simulink model "aBaja2026"  (R2025b)
settings: Solver=FixedStepAuto  StartTime=0  StopTime=1000  FixedStep=timeStep  RelTol=1e-3
PostLoadFcn:
  | helperSLTrajectoryFollowerWithRRScenarioSetup
InitFcn:
  | helperSLTrajectoryFollowerWithRRScenarioSetup
  | worldActor=rrSim.getScenario();
  | world = worldActor.actor_spec.world_spec;
  | % Inputs you already have (example):
  | EgoActorID  = 1;
  | egoSetSpeed = 0;
  | 
  | % Get world + actors
  | 
  | 
  | % --- Find the ego actor (vectorized, minimal overhead) ---
  | actorIDs = arrayfun(@(a) str2double(a.actor_runtime.id), world.actors);
  | idx = (actorIDs == EgoActorID);
  | 
  | if nnz(idx) ~= 1
  |     error("Actor with ActorID:%d does not exist (or is not unique).", EgoActorID);
  | end
  | 
  | ego = world.actors(idx);
  | 
  | % --- Build 4x4 pose matrix quickly ---
  | temp_m = ego.actor_runtime.pose.matrix;
  | pose = [temp_m.col0.x temp_m.col1.x temp_m.col2.x temp_m.col3.x; ...
  |         temp_m.col0.y temp_m.col1.y temp_m.col2.y temp_m.col3.y; ...
  |         temp_m.col0.z temp_m.col1.z temp_m.col2.z temp_m.col3.z; ...
  |         temp_m.col0.w temp_m.col1.w temp_m.col2.w temp_m.col3.w];
  | 
  | rotm = pose(1:3,1:3);
  | pos  = pose(1:3,4)';   % [x y z] meters
  | 
  | % --- Euler angles from rotation matrix (ZYX: yaw, pitch, roll) ---
  | % If you have Robotics System Toolbox, rotm2eul exists; otherwise keep internal.
  | if exist("rotm2eul","file")
  |     eulZYX = rotm2eul(rotm,"ZYX");                 % radians: [yaw pitch roll]
  | else
  |     eulZYX = robotics.internal.rotm2eul(rotm,"ZYX");% radians: [yaw pitch roll]
  | end
  | 
  | % RoadRunner yaw -> conventional yaw:
  | yawDeg   = rad2deg(eulZYX(1)) + 90;
  | yawDeg   = mod(yawDeg + 180, 360) - 180;           % wrap to (-180,180]
  | pitchDeg = rad2deg(eulZYX(2));
  | rollDeg  = rad2deg(eulZYX(3));
  | 
  | % --- (Optional) reproduce your actorPose struct (kept consistent) ---
  | vGlobal = [egoSetSpeed*cosd(yawDeg), egoSetSpeed*sind(yawDeg), 0];
  | vBody   = (rotm' * vGlobal')';                      % body-fixed velocity
  | 
  | actorPose = struct( ...
  |     'ActorID', double(EgoActorID), ...
  |     'Position', pos, ...
  |     'Velocity', vGlobal, ...
  |     'vehicleFrameVelocity', [vBody(2), -vBody(1), vBody(3)], ...
  |     'Roll',  rollDeg, ...
  |     'Pitch', pitchDeg, ...
  |     'Yaw',   yawDeg, ...
  |     'AngularVelocity', [0 0 0]);
  | 
  | % --- Inline replacement for poseToSim3DInputs ---
  | % IMPORTANT: your original poseToSim3DInputs uses radians (pi terms),
  | ... (+13 lines)
undefined symbols (not defined in the file): Defined, Ego, egoPathWidth, Lane, m, matlabshared, n, Pose, Sim3dSensor, timeStep, trackPosSelector, User, Velocity
libraries: roadrunnerscenario x9, drivingvehiclecontroller x3, simulink_extras x3, sim3dautolib x2, drivingscenarioandsensors x1, sim3dcameralib x1, sim3dlib x1, simulink x1
(part 2 of 2)

== matlab function aBaja2026/Subsystem/AEB Controller/Find MIO ==
  data: confirmedTracks input size=[1 1]; x output size=[1 1]; vx output size=[1 1]; positionSelector input; laneWidth input; relativeYawAngle output double size=[1 1]; egoSpeed input double size=[1 1]
function [x,vx, relativeYawAngle] = findMIO(confirmedTracks, positionSelector, laneWidth, egoSpeed)
% This function finds the lead car: a car in front of the ego car that
% satisfies all the criteria below:
% * Within the ego car's lane.
% * In front of the ego car.
% * Closest to the ego car.

% Important notes:
% 1. If you change state definition, change the following:
%       State = [x;vx;y;vy;z;vz] (3D constant velocity)
numStates = 6;
relativeYawAngle =0 ;
% 2. The ego car is assumed to be traveling in the middle of its lane.
halfLaneWidth = laneWidth/2;

% Initialize outputs and parameters
maxX = cast(1000, 'like', confirmedTracks.Tracks(1).State);  % Far enough forward so that no track is expected to exceed this distance
trackID = 0;
crossingTargetLateralDist = 18;
targetCollisionThresholdTime = 2; % Collision threshold time beyond which the target should be treated as MIO 
stationaryVelocityThreshold = eps('single'); % Threshold to determine if a target is effectively stationary relative to the world

for i = 1:confirmedTracks.NumTracks
    position = positionSelector * confirmedTracks.Tracks(i).State;
    x = position(1); % Longitudinal position of the track relative to ego
    y = position(2); % Lateral position of the track relative to ego

    if x < maxX && x > 0 % No point checking otherwise
        % Detect cross target as MIO to avoid collision
        
        if (-crossingTargetLateralDist <= y) && (y <= crossingTargetLateralDist) &&  ...
                abs(norm([confirmedTracks.Tracks(i).State(2), confirmedTracks.Tracks(i).State(4), confirmedTracks.Tracks(i).State(6)]) - egoSpeed) >= stationaryVelocityThreshold
            estimatedCollisionTime = confirmedTracks.Tracks(i).State(1)/abs(confirmedTracks.Tracks(i).State(2));
            if(targetCollisionThresholdTime>abs(estimatedCollisionTime))
                maxX = x;
                trackID = i;
            end
        end

        yleftLane  = polyval([0, 0,  halfLaneWidth],x); % Half a lane to the left
        yrightLane = polyval([0, 0, -halfLaneWidth],x); % Half a lane to the right
        % Find a new lead car
        if (yrightLane <= y) && (y <= yleftLane)
            maxX = x;
            trackID = i;
        end
    end
end

if trackID>0
    mioState = confirmedTracks.Tracks(trackID).State;
    relativeYawEgoFrame = atan2(mioState(4), mioState(2));
    relativeYawAngle = relativeYawEgoFrame;
else
    mioState = zeros(numStates,1,'like',confirmedTracks.Tracks(1).State);
    mioState(1) = 500;
    mioState(2) = 0.01;
end

% Output:
x = mioState(1);    % Longitudinal position of the lead car
vx = mioState(2);   % Longitudinal velocity of the lead car

== matlab function aBaja2026/Subsystem/MATLAB Function ==
  data: u input; y output
function y = fcn(u)

y = norm(u);

== matlab function aBaja2026/Subsystem2/Pack Actor Pose/Pose Generation ==
  data: pose input; currPose output
function currPose = generatePose(pose)

yaw = deg2rad(pose(3));
rotm = eul2rotm([yaw 0 0]);

currPose = [[rotm [pose(1:2) 0]']; [0 0 0 1]];
